simulink model "PHIL_Simulation"  (R2025a)
settings: Solver=ode23t  StartTime=0.0  StopTime=1.5  FixedStep=0.001  MaxStep=1e-5  RelTol=1e-3
PostLoadFcn:
  | if any(exist('dsrtsu_mdlpostloadfcn', 'file') ~= 0), dsrtsu_mdlpostloadfcn('Execute', bdroot); end
InitFcn:
  | , if any(exist('rtifpga_mdlclblib', 'file') ~= 0), rtifpga_mdlclblib('Init', bdroot); end,
  | , if any(exist('dsmpb_private', 'file') ~= 0), dsmpb_private('dsmpb_mdlclblib', 'Init', bdroot); end,
libraries: fl_lib x5, nesl_utility x4, ee_lib x2, spsPWMGeneratorDCDCLib x1
PreSaveFcn:
  | , if any(exist('dsmpb_private', 'file') ~= 0), dsmpb_private('dsmpb_mdlclblib', 'PreSave', bdroot); end,
CloseFcn:
  | , if any(exist('dsmpb_private', 'file') ~= 0), dsmpb_private('dsmpb_mdlclblib', 'Close', bdroot); end,
settings Model: DSRTSU_INTERNAL_RTIFPGA=220  DSRTSU_INTERNAL_RTISTBM_VER=25.1  Creator=e94179u  LastModifiedBy=e94179u
settings OptimizationCC: BlockReduction=off  ConditionallyExecuteInputs=off  OptimizeBlockIOStorage=off  BufferReuse=off
settings DebuggingCC: TasksWithSamePriorityMsg=none
settings HardwareCC: ProdBitPerLong=64.0  ProdLargestAtomicInteger=Integer  ProdWordSize=32.0  ProdLongLongMode=on  ProdHWDeviceType=Custom Processor->Custom
settings ModelReferenceCC: EnableParallelModelReferenceBuilds=on
settings RTWCC: SystemTargetFile=dsrt.tlc  GenCodeOnly=on  MakeCommand=make_dsrt  TemplateMakefile=dsrt_default_tmf  RTWVerbose=off  Description=dSPACE Target DSRT - Generates SIC files for import by ConfigurationDesk and VEOS. Provides code generation for Simulink models imported in ConfigurationDesk.
settings STFCustomTargetCC: SystemTargetFile=dsrt.tlc  TargetLangStandard=C99 (ISO)  MultiwordLength=2048.0  DynamicStringBufferSize=256.0  ParMdlRefBuildCompliant=on  GRTInterface=off  DSTargetArchitecture=Default  TRCGenerateVirtualBlocks=off  TRCGenerateDerivatives=off  TRCGenerateLabels=off  VDFType=TRC  TRCGenerateStates=off  TRCIsOmitVdOn=on  TRCOnlyGlobals=off  TRCGenerateParamValues=off
settings GRTTargetCC: CompOptLevelCompliant=off  ConcurrentExecutionCompliant=off  CombineOutputUpdateFcns=off  MatFileLogging=off  CPPClassGenCompliant=off  UseToolchainInfoCompliant=off

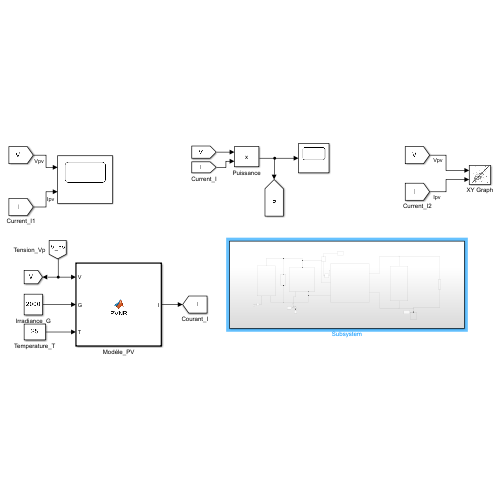
[thumbnail: Simulink's stored preview of the top-level diagram]
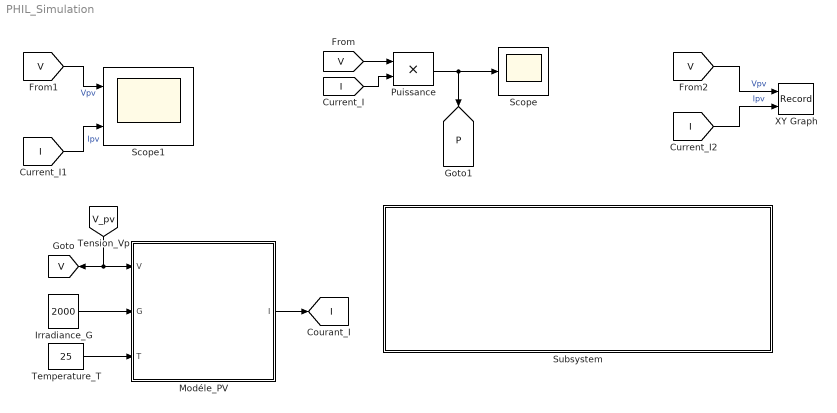
== system PHIL_Simulation ==
  Irradiance_G : Constant  Value=2000
  Modéle_PV : MATLAB Function  TreatAsAtomicUnit=on
  Puissance : Product
  Scope : Scope
      settings: ActiveDisplayYMinimum=-31.070508181508981  ActiveDisplayYMaximum=279.63457363358089
  Scope1 : Scope  NumInputPorts=2
      settings: ActiveDisplayYMinimum=-5.7530332301237044  ActiveDisplayYMaximum=40.727435180796526
  Subsystem : Subsystem
  Temperature_T : Constant  Value=25
  XY Graph : Record  NumPorts=2.0  FileSettingsInternal="{\"entries\":[{\"content\":{\"excelSettings\":{\"content\":{},\"type\":\"Streamout.ExcelSettings\"},\"parquetSettings\":{\"content\":{},\"type\":\"Streamout.ParquetSettings\"}},\"type\":\"Streamout.FileSettingStorage\",\"uuid\":\"\"}],\"packageUris\":[\"http:\\/\\/schema.mathworks.com\\/mf0\\/streamout_blocks\\/R2020a\"],\"version\":\"1.0\"}"  FrameSettings=[0, 0]  Layout=[1 1]  SignalsInternal="{\"entries\":[{\"content\":{\"signals\":[{\"content\":{\"blockPath\":[],\"dimensions\":[1],\"domain\":\"\",\"lineColor\":\"#a2142f\",\"plots\":[ 1 ],\"port\":1,\"sid\":[\"\"],\"signalID\":1,\"signalName\":\"Vpv\"},\"type\":\"RecordBlkView.Signal\",\"uuid\":\"\"},{\"content\":{\"blockPath\":[],\"dimensions\":[1],\"domain\":\"\",\"lineColor\":\"#139fff\",\"plots\":[ 1 ],\"port\":2,\"sid\":[\"\"],\"signalID\":2,\"signalName\":\"Ipv\"},\"type\":\"RecordBlkView.Signal\",\"uuid\":\"\"}]},\"type\":\"RecordBlkView.InputSignals\",\"uuid\":\"\"}],\"packageUris\":[\"http:\\/\\/schema.mathworks.com\\/mf0\\/streamout_blocks\\/R2020a\"],\"version\":\"1.0\"}"  VisualizationBindings="{\"xyplotplugin\":{\"info\":[{\"series\":[{\"bindingParametersList\":[{\"parameter\":\"X-Axis\",\"signalID\":1,\"signalName\":\"Vpv\"},{\"parameter\":\"Y-Axis\",\"signalID\":2,\"signalName\":\"Ipv\"}],\"seriesID\":0}],\"subplotID\":1}]}}"  CompatibilityTag=XY
  tag scope: I=global, P=global, V=global
  wires:
  [V] -> Puissance/1
  Puissance/1 -> Scope/1, [P]
  [I] -> Puissance/2
  [V_pv] -> [V], Modéle_PV/1(V)
  Temperature_T/1 -> Modéle_PV/3(T)
  Irradiance_G/1 -> Modéle_PV/2(G)
  Modéle_PV/1(I) -> [I]
  [I] -> Scope1/2  "Ipv"
  [V] -> Scope1/1  "Vpv"
  [I] -> XY Graph/2  "Ipv"
  [V] -> XY Graph/1  "Vpv"

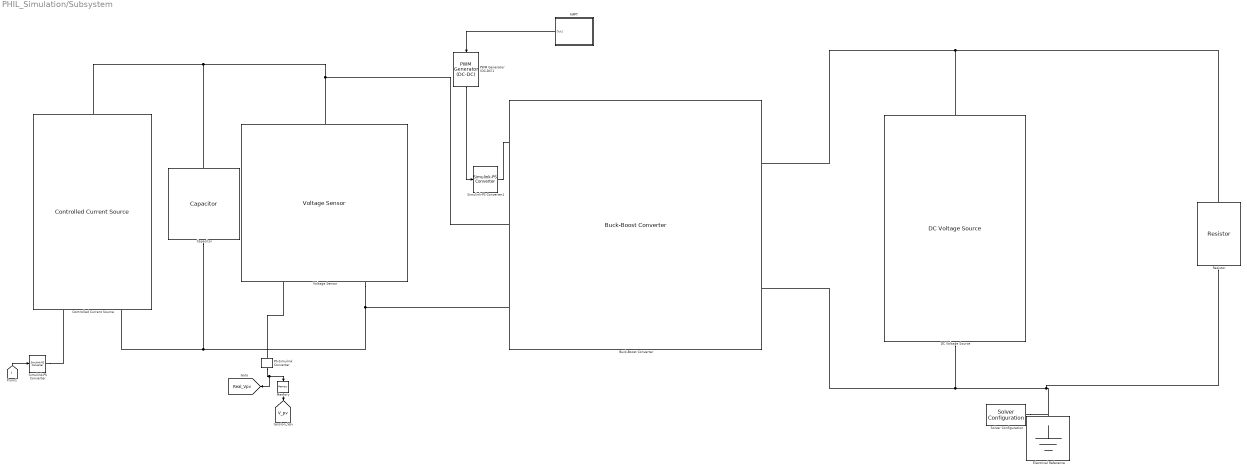
== system PHIL_Simulation/Subsystem ==
  Buck-Boost Converter : ee_lib/Semiconductors & Converters/Converters/Buck-Boost Converter  port_option=ee.enum.controlport.ps  device_type=ee.enum.converters.switchingdevice.ideal  Vf=0.8 V  Ron=0.001 Ohm  Rds=0.001 Ohm  Goff=1e-5 1/Ohm  Vgt=1 V  Vgt_off=-1 V  Ih=1 A  Vth=0.5 V  K=0  diode_param=ee.enum.converters.diode.nodynamics  diode_Vf=0.8 V  diode_Ron=0.001 Ohm  diode_Goff=1e-5 1/Ohm  diode_C=50 nF  diode_iRM=-235 A  diode_iF=300 A  diode_idot=-50 A/us  diode_trr_param=ee.enum.converters.diodetrr.trr_factor  diode_trr_factor=3  diode_trr=15 us  diode_Qrr=1500 s*uA  Lf=1e-3 H  Rl=0 Ohm  Cf=100e-6 F  Rf=0.01 Ohm  snubber_type=ee.enum.converters.snubber.exclude  Cs=1e-7 F  Rs=0.1 Ohm  iL_specify=on  iL_priority=High  iL=0 A  iL_nominal_specify=off  iL_nominal_value=1  iL_nominal_unit=A  vc_specify=on  vc_priority=High  vc=0 V  vc_nominal_specify=off  vc_nominal_value=1  vc_nominal_unit=V
      settings: InternalSimscapePortConfiguration="{\"Bottom\":[],\"Left\":[{\"id\":\"G\",\"label\":\"G\",\"type\":\"input\"},{\"id\":\"p1\",\"label\":\"1+\",\"type\":\"foundation.electrical.electrical\"},{\"id\":\"n1\",\"label\":\"1-\",\"type\":\"foundation.electrical.electrical\"}],\"Right\":[{\"id\":\"p2\",\"label\":\"2+\",\"type\":\"foundation.electrical.electrical\"},{\"id\":\"n2\",\"label\":\"2-\",\"type\":\"foundation.electrical.electrical\"}],\"Top\":[]}"
  Capacitor : fl_lib/Electrical/Electrical Elements/Capacitor  c=1e-3 F  r=1e-6 Ohm  g=0 1/Ohm  i_specify=off  i_priority=None  i=0 A  i_nominal_specify=off  i_nominal_value=1  i_nominal_unit=A  v_specify=off  v_priority=None  v=0 V  v_nominal_specify=off  v_nominal_value=1  v_nominal_unit=V  vc_specify=on  vc_priority=High  vc=36 V  vc_nominal_specify=off  vc_nominal_value=1  vc_nominal_unit=V
  Controlled Current Source : fl_lib/Electrical/Electrical Sources/Controlled Current Source
  DC Voltage Source : ee_lib/Additional Components/SPICE Sources/DC Voltage Source  DC=-50 V
  Electrical Reference : fl_lib/Electrical/Electrical Elements/Electrical Reference
  MPPT : Subsystem
  Memory : Memory  InitialCondition=30
  PS-Simulink Converter : nesl_utility/PS-Simulink Converter  PhysicalDomain=network_engine_domain  SubClassName=ps_output  LeftPortType=input  RightPortType=output  PseudoPeriodic=off  Frequencies=[]  VectorFormat=inherit  Unit=inherit  AffineConversion=off
  PWM Generator (DC-DC)1 : spsPWMGeneratorDCDCLib/PWM Generator (DC-DC)  Fsw=10000  Ts=1e-6
  Resistor : fl_lib/Electrical/Electrical Elements/Resistor  R=50 Ohm  i_specify=off  i_priority=None  i=0 A  i_nominal_specify=off  i_nominal_value=1  i_nominal_unit=A  v_specify=off  v_priority=None  v=0 V  v_nominal_specify=off  v_nominal_value=1  v_nominal_unit=V
  Simulink-PS Converter : nesl_utility/Simulink-PS Converter  PhysicalDomain=network_engine_domain  SubClassName=ps_input  LeftPortType=input  RightPortType=output  PseudoPeriodic=off  Frequencies=[]  NoiseDistribution=none  NoiseParameters=[]  Unit=1  AffineConversion=off  FilteringAndDerivatives=provide  SimscapeFilterOrder=1  InputFilterTimeConstant=0.001  UdotUserProvided=0
  Simulink-PS Converter1 : nesl_utility/Simulink-PS Converter  PhysicalDomain=network_engine_domain  SubClassName=ps_input  LeftPortType=input  RightPortType=output  PseudoPeriodic=off  Frequencies=[]  NoiseDistribution=none  NoiseParameters=[]  Unit=1  AffineConversion=off  FilteringAndDerivatives=provide  SimscapeFilterOrder=1  InputFilterTimeConstant=0.001  UdotUserProvided=0
  Solver Configuration : nesl_utility/Solver Configuration  PhysicalDomain=network_engine_domain  SubClassName=solver  LeftPortType=input  RightPortType=generic  Tones=[]  Harmonics=[]  SimulateNoise=off  Profile=off  UseLocalSampling=off  EnableSwitchedLinearOptims=on  FrequencyDomain=off  UseCCode=off  RelTol=0.001  AbsTol=0.001  MinStep=1e-09  ToWorkspace=off  RevertToSquareIcSolve=off  NumHomotopyIterations=100  PhasorMode=off  PhasorModeNumHarmonics=1  ConsistencySolver=NEWTON_XTOL_AFTER_FTOL  IndexReductionMethod=DerivativeReplacement  DoDC=off  ResidualTolerance=1e-09  ConsistencyTolSource=GLOBAL  ConsistencyAbsTol=0.001  ConsistencyRelTol=0.001  ConsistencyTolFactor=0.001  UseLocalSolver=off  LocalSolverChoice=NE_BACKWARD_EULER_ADVANCER  ResolveIndetEquations=on  FunctionEvalNumThread=1  LocalSolverSampleTime=0.001  DoFixedCost=off  MaxNonlinIter=3  MaxModeIter=2  ComputeImpulses=off  ImpulseIterations=2  LinearAlgebra=auto  LinearAlgebraNumThread=0  EquationFormulation=NE_TIME_EF  DelaysMemoryBudget=1024  AutomaticFiltering=on  FilteringTimeConstant=0.001  PartitionStorageMethod=AS_NEEDED  PartitionMemoryBudget=1024  PartitionMethod=ROBUST  MultibodyUseLocalSolver=off  MultibodyLocalSolverChoice=ODE1  MultibodyLocalSolverSampleTime=0.001
  Voltage Sensor : fl_lib/Electrical/Electrical Sensors/Voltage Sensor
  tag scope: Real_Vpv=global, V_pv=global
  wires:
  [I] -> Simulink-PS Converter/1
  PS-Simulink Converter/1 -> Memory/1, [Real_Vpv]
  Memory/1 -> [V_pv]
  PWM Generator (DC-DC)1/1 -> Simulink-PS Converter1/1
  MPPT/1(Out1) -> PWM Generator (DC-DC)1/1
  connections:
  Simulink-PS Converter/RConn1 -- Controlled Current Source/RConn1
  Controlled Current Source/LConn1 -- Capacitor/LConn1 -- Voltage Sensor/LConn1 -- Buck-Boost Converter/LConn2
  Buck-Boost Converter/LConn3 -- Voltage Sensor/RConn2 -- Capacitor/RConn1 -- Controlled Current Source/RConn2
  Simulink-PS Converter1/RConn1 -- Buck-Boost Converter/LConn1
  Solver Configuration/RConn1 -- Electrical Reference/LConn1 -- Resistor/RConn1 -- DC Voltage Source/RConn1 -- Buck-Boost Converter/RConn2
  Resistor/LConn1 -- DC Voltage Source/LConn1 -- Buck-Boost Converter/RConn1
  PS-Simulink Converter/LConn1 -- Voltage Sensor/RConn1

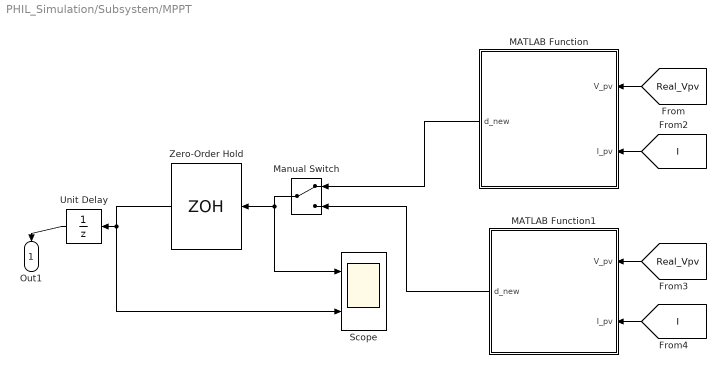
== system PHIL_Simulation/Subsystem/MPPT ==
  MATLAB Function : MATLAB Function  TreatAsAtomicUnit=on
  MATLAB Function1 : MATLAB Function  TreatAsAtomicUnit=on
  Manual Switch : ManualSwitch
  Scope : Scope  NumInputPorts=2
      settings: ActiveDisplayYMinimum=0.60866800366543694  ActiveDisplayYMaximum=0.61280432355106762  DataLoggingVariableName=ScopeData2
  Unit Delay : UnitDelay  InitialCondition=0.75  SampleTime=-1  HasFrameUpgradeWarning=on
  Zero-Order Hold : ZeroOrderHold  SampleTime=-1
  Out1 : Outport
  wires:
  [Real_Vpv] -> MATLAB Function/1(V_pv)
  [I] -> MATLAB Function1/2(I_pv)
  Manual Switch/1 -> Scope/1, Zero-Order Hold/1
  Zero-Order Hold/1 -> Scope/2, Unit Delay/1
  Unit Delay/1 -> Out1/1
  [Real_Vpv] -> MATLAB Function1/1(V_pv)
  [I] -> MATLAB Function/2(I_pv)
  MATLAB Function/1(d_new) -> Manual Switch/1
  MATLAB Function1/1(d_new) -> Manual Switch/2

== matlab function PHIL_Simulation/Subsystem/MPPT/MATLAB Function ==
  settings: updateMethod=DISCRETE  sampleTime=0.01
  data: V_pv input; I_pv input; d_new output
function d_new = MPPT_intuitif(V_pv, I_pv)
    persistent V_old P_old
    
    if isempty(V_old)
        V_old = 20;     
        P_old = 0;
    end
    
    V_bus = 50;
    D = 0.00001;            
    
    % Puissance actuelle
    P_now = V_pv * I_pv;
    
    % Variations depuis l'itération précédente
    dP = P_now - P_old;
    dV = V_pv - V_old;
    
    % Logique de Baghli : décide V_new
    if dP > 0
        if dV > 0
            V_new = V_pv + D;
        else
            V_new = V_pv - D;
        end
    else
        if dV < 0
            V_new = V_pv + D;
        else
            V_new = V_pv - D;
        end
    end
    
    % Sécurité sur V_new
    if V_new < 1
        V_new = 1;
    end
    if V_new > 36
        V_new = 36;
    end
    
    % Conversion V_new → duty cycle (formule buck-boost)
    d_new = V_bus / (V_bus + V_new);
    
    % Saturation duty
    if d_new < 0.1
        d_new = 0.1;
    end
    if d_new > 0.9
        d_new = 0.9;
    end
    
    % Mémorisation pour le prochain appel
    V_old = V_pv;
    P_old = P_now;
end

== matlab function PHIL_Simulation/Modéle_PV ==
  data: V input; I output; G input; T input
function I = PVNR(V, G, T)
    
    T = T + 273.15;       % conversion en Kelvin
    V = V / 60;           % tension par cellule
    
    % Paramètres panneau 250W
    Isc = 8.69;
    Voc = 0.61;
    Kv = -0.0038;
    Ki = 0.004;
    Ns = 60;
    k = 1.3806503e-23;
    q = 1.60217646e-19;
    a = 1.3;
    Rs = 0.04/60;
    Rp = 1271.1/60;
    Gn = 1000;
    Tn = 298.15;
    dT = T - Tn;
    
    % Photocourant et courant de saturation
    Vt = k*T/q;
    Io = (Isc + Ki*dT) / (exp(q*(Voc + Kv*dT)/(a*k*Tn)) - 1);
    Iph = (Isc + Ki*dT) * G/Gn;
    
    % Newton-Raphson borné à 50 itérations
    I = 4;  
    for iter = 1:50
        g = Iph - Io*(exp(q*(V + I*Rs)/(k*T*a)) - 1) - (V + I*Rs)/Rp - I;
        glin = -Io*q*Rs/(k*T*a) * exp(q*(V + I*Rs)/(k*T*a)) - Rs/Rp - 1;
        
        if abs(g) < 0.001
            break;
        end
        if glin ~= 0
            I = I - g/glin;
        else
            break;
        end
    end
    
    if I < 0
        I = 0;
    end
end

== matlab function PHIL_Simulation/Subsystem/MPPT/MATLAB Function1 ==
  settings: updateMethod=DISCRETE  sampleTime=0.01
  data: V_pv input; I_pv input; d_new output
function d_new = MPPT_Optimise(V_pv, I_pv)
    % On ajoute V_ref à la mémoire de l'algorithme
    persistent V_ref V_old P_old
    
    if isempty(V_ref)
        V_ref = 20; 
        V_old = 20;     
        P_old = 0;
    end
    
    V_bus = 50;
    D = 0.1; 
    
    P_now = V_pv * I_pv;
    dP = P_now - P_old;
    dV = V_pv - V_old; 
    
    
    if dP > 0
        if dV > 0
            V_ref = V_ref + D;
        else
            V_ref = V_ref - D;
        end
    else
        if dV < 0
            V_ref = V_ref + D;
        else
            V_ref = V_ref - D;
        end
    end
    
    if V_ref < 10
        V_ref = 10;
    end
    if V_ref > 36
        V_ref = 36;
    end
    
    
    d_new = V_bus / (V_bus + V_ref);
    
    if d_new < 0.1
        d_new = 0.1;
    end
    if d_new > 0.9
        d_new = 0.9;
    end
    
    V_old = V_pv;
    P_old = P_now;
end
